simulink model "MFTest"  (R2019a)
settings: Solver=VariableStepAuto  StartTime=0.0  StopTime=10.0  RelTol=1e-3
settings Model: Creator=Administrator  LastModifiedBy=Administrator

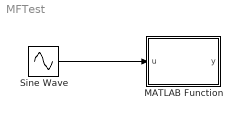
== system MFTest ==
  MATLAB Function : MATLAB Function  TreatAsAtomicUnit=on
  Sine Wave : Sin  SampleTime=0
  wires:
  Sine Wave/1 -> MATLAB Function/1(u)

== matlab function MFTest/MATLAB Function ==
  data: u input; y output
function y = fcn(u)

y = [u;u-0.1;u-0.2];
